simulink model "partitionedLifitngBdy_th"  (R2018b)
settings: Solver=VariableStepAuto  StartTime=0.0  StopTime=0  RelTol=1e-3
values from neighbouring files (symbols this model uses):
  angVelBdy = [0 0 0]    [partitionedLifitngBdy_ts.m]
  euler = [0;0;0]    [partitionedLifitngBdy_ts.m]
  vCM = [0 0.0 0.0]    [partitionedLifitngBdy_ts.m]
  vFlow = [1 0 0]    [partitionedLifitngBdy_ts.m]
libraries: partitionedLifitngBdy_cl x1
settings Model: Creator=mcobb  LastModifiedBy=asiddiq2

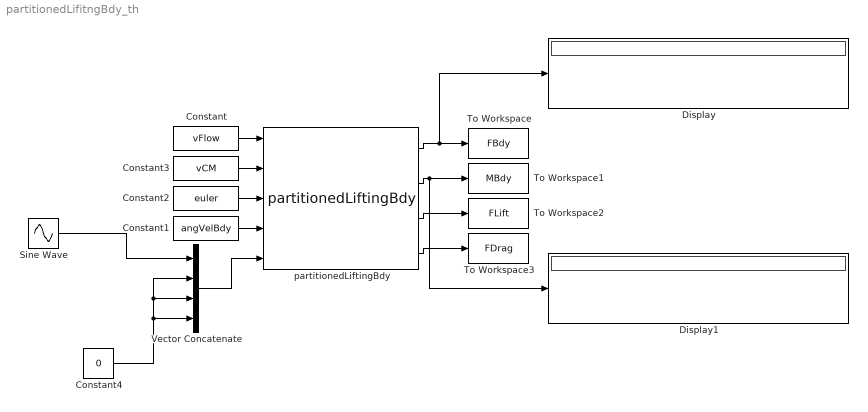
== system partitionedLifitngBdy_th ==
  Constant : Constant  Value=vFlow  VectorParams1D=off
  Constant1 : Constant  Value=angVelBdy  VectorParams1D=off
  Constant2 : Constant  Value=euler  VectorParams1D=off
  Constant3 : Constant  Value=vCM  VectorParams1D=off
  Constant4 : Constant  Value=0
  Display : Display
  Display1 : Display
  Sine Wave : Sin  Amplitude=0  SampleTime=0
  To Workspace : ToWorkspace  VariableName=FBdy  SaveFormat=Timeseries  SampleTime=-1
  To Workspace1 : ToWorkspace  VariableName=MBdy  SaveFormat=Timeseries  SampleTime=-1
  To Workspace2 : ToWorkspace  VariableName=FLift  SaveFormat=Timeseries  SampleTime=-1
  To Workspace3 : ToWorkspace  VariableName=FDrag  SaveFormat=Timeseries  SampleTime=-1
  Vector Concatenate : Concatenate  NumInputs=4
  partitionedLiftingBdy : partitionedLifitngBdy_cl/partitionedLiftingBdy  rho_fluid=fluidDensity  aero_struct=aeroStruct
  wires:
  partitionedLiftingBdy/1 -> Display/1, To Workspace/1
  Constant/1 -> partitionedLiftingBdy/1
  Constant1/1 -> partitionedLiftingBdy/4
  Constant2/1 -> partitionedLiftingBdy/3
  Sine Wave/1 -> Vector Concatenate/1
  partitionedLiftingBdy/3 -> To Workspace2/1
  partitionedLiftingBdy/4 -> To Workspace3/1
  Vector Concatenate/1 -> partitionedLiftingBdy/5
  Constant4/1 -> Vector Concatenate/4, Vector Concatenate/3, Vector Concatenate/2
  partitionedLiftingBdy/2 -> To Workspace1/1, Display1/1
  Constant3/1 -> partitionedLiftingBdy/2
